simulink model "mod_sim_VTMS"  (R2018b)
settings: Solver=FixedStepDiscrete  StartTime=0.0  StopTime=t_Simulation  FixedStep=delta_t  RelTol=1e-3
values from neighbouring files (symbols this model uses):
  P_charge = 150    [main_sim_VTMS.m]
undefined symbols (not defined in the file or in its folder): A_EMaschine_Getriebe, A_j_c, A_Stirn, Anzahl_Peltierelemente, b_Batteriepack, b_c, b_EMaschine, b_Getriebe, b_j, b_Ladegeraet, BatPara, c_W, delta_t, DiscIntNeverNeededParam, e_Fahrzeug, eta_EMaschine_Break_M_EMaschine, eta_EMaschine_Break_n_EMaschine, eta_EMaschine_Faktor_Volllast, eta_EMaschine_Table, eta_Getriebe, eta_Ladegeraet, eta_Leistungselektronik_Break_M_EMaschine, eta_Leistungselektronik_Break_n_EMaschine, eta_Leistungselektronik_Faktor_Volllast, eta_Leistungselektronik_Table, f_R, I_DT_U_Break_DT, I_DT_U_Break_U, I_DT_U_Value_I, i_Getriebe, I_max, Ladevorgang, M_EMaschine_max, m_Fahrzeug, m_Zuladung, n_Zelle, P_Nebenverbraucher, p_Zelle, Peltier_Max_Eff, Q_DT_U_Break_DT, Q_DT_U_Break_U, Q_DT_U_Value_Q, Q_Imax_DT_Break_DT, Q_Imax_DT_Value_Q, r_dynamisch, rho_Luft, s_Zelle, SOC_init, Steuerung_Kuehlerluefter, Steuerung_Pumpe, Steuerung_Ventil, switch_BP_Zyklus, T_Batteriepack_init, T_EMaschine_Getriebe_init, T_Ladegeraet_init, T_Ladegeraet_Offset, T_Leistungselektronik_init, T_Offset_Batteriepack, T_Offset_EMaschine_Getriebe, T_Offset_Leistungselektronik ... (+36)
libraries: simulink x3, simulink_extras x2
(part 2 of 5)

== system mod_sim_VTMS/Thermomanagementsystem/Schlauch ==
  Fluid_Schlauch_Output : Inport
  T_Umgebung [K] : Inport  Port=2
  v_Fahrzeug [m*s^-1] : Inport  Port=3
  Bus Creator : BusCreator  Inputs=11
  Bus Selector : BusSelector  OutputSignals=T_FinitesVolumen_Schlauch(1) [K],PV_Kuehlfluessigkeit_Schlauch(1) [m^3*s^-1],T_FinitesVolumen_Schlauch(2) [K],PV_Kuehlfluessigkeit_Schlauch(2) [m^3*s^-1],T_FinitesVolumen_Schlauch(3) [K],PV_Kuehlfluessigkeit_Schlauch(3) [m^3*s^-1],T_FinitesVolumen_Schlauch(4) [K],PV_Kuehlfluessigkeit_Schlauch(4) [m^3*s^-1],T_FinitesVolumen_Schlauch(5) [K],PV_Kuehlfluessigkeit_Schlauch(5) [m^3*s^-1],T_FinitesVolumen_Schlauch(6) [K],PV_Kuehlfluessigkeit_Schlauch(6) [m^3*s^-1],T_FinitesVolumen_Schlauch(7) [K],PV_Kuehlfluessigkeit_Schlauch(7) [m^3*s^-1],T_FinitesVolumen_Schlauch(8) [K],PV_Kuehlfluessigkeit_Schlauch(8) [m^3*s^-1],T_FinitesVolumen_Schlauch(9) [K],PV_Kuehlfluessigkeit_Schlauch(9) [m^3*s^-1],T_FinitesVolumen_Schlauch(10) [K],PV_Kuehlfluessigkeit_Schlauch(10) [m^3*s^-1],T_FinitesVolumen_Schlauch(11) [K],PV_Kuehlfluessigkeit_Schlauch(11) [m^3*s^-1]
  Schlauch thermisch : Subsystem
  Schlauch_Output : Outport
  wires:
  Bus Creator/1 -> Schlauch_Output/1
  Fluid_Schlauch_Output/1 -> Bus Selector/1

== system mod_sim_VTMS/Thermomanagementsystem/Wärmetauscher ==
  Fluid_Waermetauscher_Output : Inport
  T_Umgebung [K] : Inport  Port=2
  v_Fahrzeug [m*s^-1] : Inport  Port=3
  Bus Creator : BusCreator  Inputs=2
  Bus Selector : BusSelector  OutputSignals=T_FinitesVolumen_Waermetauscher(1_1) [K],PV_Kuehlfluessigkeit_Waermetauscher(1_1) [m^3*s^-1],T_FinitesVolumen_Waermetauscher(2_1) [K],PV_Kuehlfluessigkeit_Waermetauscher(2_1) [m^3*s^-1]
  Waermetauscher thermisch : Subsystem
  Waermetauscher_Output : Outport
  wires:
  Bus Creator/1 -> Waermetauscher_Output/1
  Fluid_Waermetauscher_Output/1 -> Bus Selector/1

== system mod_sim_VTMS/Thermomanagementsystem/switch_BP_Zyklus ==
  Rad_Output_Zyklus : Inport
  v_Fahrzeug_Zyklus [m/s] : Inport  Port=2
  Rad_Output_BP : Inport  Port=3
  v_Fahrzeug_BP [m/s] : Inport  Port=4
  Constant : Constant  Value=switch_BP_Zyklus
  Switch : Switch  Criteria=u2 ~= 0
  Switch1 : Switch  Criteria=u2 ~= 0
  v_Fahrzeug [m*s^-1] : Outport
  Rad_Output : Outport  Port=2
  wires:
  Constant/1 -> Switch/2, Switch1/2
  Switch1/1 -> v_Fahrzeug [m*s^-1]/1
  Switch/1 -> Rad_Output/1
  v_Fahrzeug_BP [m/s]/1 -> Switch1/1
  v_Fahrzeug_Zyklus [m/s]/1 -> Switch1/3
  Rad_Output_Zyklus/1 -> Switch/3
  Rad_Output_BP/1 -> Switch/1

== system mod_sim_VTMS/Thermomanagementsystem/Batteriepack/Abbruch, wenn SOC <= 0 ==
  SOC_Batteriepack [-] : Inport
  Relational Operator : RelationalOperator  Operator=<=  OutDataTypeStr=boolean  RndMeth=Simplest
  SoC_min [-] : Constant  Value=0
  Stop Simulation : Stop
  wires:
  SoC_min [-]/1 -> Relational Operator/2
  Relational Operator/1 -> Stop Simulation/1
  SOC_Batteriepack [-]/1 -> Relational Operator/1

== system mod_sim_VTMS/Thermomanagementsystem/Batteriepack/Batteriepack(1) elektrisch ==
  note: -> Annahme: Das Batteriepack besteht aus komplett identischen Zellen
      | -> Annahme: Das Batteriepack besteht aus NCR18650PF-Zellen (zylindrische Lithium-Ionen-Zelle)
      | -> Deswegen ist das Batteriepack derart modelliert, dass dass nur eine Zelle elektrisch berechnet wird und basierend auf den resultierenden Zellgrößen die Batteriepackgrößen bestimmt werden
      | -> Dazu ist ein Zellmodell aus dem am FTM vorhandenen Batteriepackmodell, das im Rahmen der Semesterarbeit "Modellbasierte Entwicklung eines vollparametrischen Batteriepackmodells für Elektro- und Hybridfahrzeuge" entwickelt wurde, abgeleitet
      |
      | -> Die Strombelastung einer Zelle wird aus der Leistungsanforderung an eine Zelle und der Klemmenspannung einer Zelle berechnet
      | -> E ine positive Leistungsanforderung an eine Zelle führt zu deren Entladung
      | -> Im Batteriepackmodell bzw. im daraus abgeleiteten Zellmodell sind Entladeströme negativ definiert
      | -> Deswegen wird bei der Berechnung der Strombelastung einer Zelle mit -1 multipliziert, um bei einer positiven Leistungsanforderung an eine Zelle korrekterweise eine negative Strombelastung einer Zelle zu erhalten
      | -> Das Zellmodell berechnet zu einem Auswertungszeitpunkt basierend auf der Strombelastung einer Zelle die Klemmenspannung einer Zelle
      | -> Deswegen muss bei der Berechnung der Strombelastung einer Zelle die Klemmenspannung einer Zelle vom vorherigen Auswertungszeitpunkt verwendet werden
      | -> Dadurch wird ein Fehler gemacht, der wegen der zeitdiskreten Auswertung jedoch nicht vermeidbar ist
      | -> Zu Beginn der Simulation wird statt der Klemmenspannung einer Zelle vom vorherigen Auswertungszeitpunkt das initiale Potential einer Zelle herangezogen
      | -> U_Potential_init = U_SOC_init + U_Hysterese_init + U_RC1_init + U_RC2_init
      |
      | P_Zelle = P_Batteriepack / n_Zelle
      | mit n_Zelle = p_Zelle * s_Zelle
      |
      | I_Zelle = - P_Zelle / U_Zelle
  note: -> Das Batteriepackmodell basiert auf Temperaturen in °C statt in K
      |
      | -> Das Batteriepack wird als Blockkapazität betrachtet
      | -> Temperatur des Batteriepacks = Temperatur jeder Zelle
  T_Batteriepack [K] : Inport
  P_Batteriepack [W] : Inport  Port=2
  Add : Sum  Inputs=++++
  Batteriepackgrößen : Subsystem
  Constant : Constant  Value=SOC_init  VectorParams1D=off
  Constant1 : Constant  Value=U_Hysterese_init  VectorParams1D=off
  Constant2 : Constant  Value=U_RC1_init  VectorParams1D=off
  Constant3 : Constant  Value=U_RC2_init  VectorParams1D=off
  Constant4 : Constant  Value=n_Zelle  VectorParams1D=off
  Constant5 : Constant  Value=273.15  VectorParams1D=off
  Delay : Delay  DelayLength=1  InitialConditionSource=Input port  InitialCondition=0
      settings: InputPortMap=u0,p4
  Divide : Product  Inputs=*/
  Divide1 : Product  Inputs=*/
  Gain : Gain  Gain=-1
  SOC --> U_SOC : Lookup_n-D  NumberOfTableDimensions=1  BreakpointsForDimension1=BatPara.ECMPara.OCV.Steps.SOC_ch  BreakpointsForDimension2=[1:3]  IndexSearchMethod=Linear search  BeginIndexSearchUsingPreviousIndexResult=on  Table=BatPara.ECMPara.OCV.Steps.U_mean  ExtrapMethod=Clip  RemoveProtectionInput=on  UseLastTableValue=on  RndMeth=Simplest  InputSameDT=on
  Subtract : Sum  Inputs=+-
  "Zellmodell (abgeleitet aus Batteriepackmodell -> siehe FTM)" : Subsystem  TreatAsAtomicUnit=on
  I_Batteriepack [A] : Outport
  U_Batteriepack [V] : Outport  Port=2
  SOC_Batteriepack [-] : Outport  Port=3
  eta_Batteriepack [%] : Outport  Port=4
  P_Verlust_Batteriepack [W] : Outport  Port=5
  wires:
  Batteriepackgrößen/4(eta_Batteriepack [%]) -> eta_Batteriepack [%]/1
  Batteriepackgrößen/2(U_Batteriepack [V]) -> U_Batteriepack [V]/1
  Batteriepackgrößen/1(I_Batteriepack [A]) -> I_Batteriepack [A]/1
  Constant5/1 -> Subtract/2
  Subtract/1 -> "Zellmodell (abgeleitet aus Batteriepackmodell -> siehe FTM)"/2(T_Zelle [°C])
  "Zellmodell (abgeleitet aus Batteriepackmodell -> siehe FTM)"/4(P_Verlust_Zelle_reversibel [W]) -> Batteriepackgrößen/6(P_Verlust_Zelle_reversibel [W])
  Add/1 -> Delay/2
  "Zellmodell (abgeleitet aus Batteriepackmodell -> siehe FTM)"/1(U_Zelle [V]) -> Batteriepackgrößen/3(U_Zelle [V]), Delay/1
  Delay/1 -> Divide1/2  "U_Zelle [V]"
  SOC --> U_SOC/1 -> Add/1
  Constant/1 -> SOC --> U_SOC/1
  Divide1/1 -> Gain/1
  Constant1/1 -> Add/2
  Constant4/1 -> Divide/2
  "Zellmodell (abgeleitet aus Batteriepackmodell -> siehe FTM)"/3(P_Verlust_Zelle_irreversibel [W]) -> Batteriepackgrößen/5(P_Verlust_Zelle_irreversibel [W])
  Divide/1 -> Divide1/1, Batteriepackgrößen/1(P_Zelle [W])  "P_Zelle [W]"
  P_Batteriepack [W]/1 -> Divide/1
  Constant2/1 -> Add/3
  Batteriepackgrößen/5(P_Verlust_Batteriepack [W]) -> P_Verlust_Batteriepack [W]/1
  T_Batteriepack [K]/1 -> Subtract/1
  Constant3/1 -> Add/4
  Gain/1 -> "Zellmodell (abgeleitet aus Batteriepackmodell -> siehe FTM)"/1(I_Zelle [A]), Batteriepackgrößen/2(I_Zelle [A])
  "Zellmodell (abgeleitet aus Batteriepackmodell -> siehe FTM)"/2(SOC_Zelle [-]) -> Batteriepackgrößen/4(SOC_Zelle [-])
  Batteriepackgrößen/3("SOC_Batteriepack [-] ") -> SOC_Batteriepack [-]/1

== system mod_sim_VTMS/Thermomanagementsystem/Batteriepack/Batteriepack(1) thermisch ==
  note: T_Batteriepack_k+1 = T_Batteriepack_k + delta_T_Batteriepack für k = Auswertungszeitpunkt
      | = T_Batteriepack_k + b_Batteriepack * (P_Verlust_Batteriepack_k - PQ_Batteriepack_k) für k = Auswertungszeitpunkt
      |
      | mit b_Batteriepack = delta_t / C_Batteriepack
  note: -> Das Batteriepack wird als Blockkapazität aufgefasst und wird nicht als Zusammenschluss einzelner Zellen betrachtet
      |
      | -> Das Batteriepack besitzt eine eigene Temperatur und wird als diabat zu seiner Umgebung betrachtet
      | -> Es gibt also einen Wärmeaustausch zwischen Batteriepack und Umgebungsluft
      | -> Zudem gibt es einen Wärmeaustausch zwischen Batteriepack und Kühlflüssigkeit
      | -> Das Batteriepack besitzt eine Verlustleistung
  P_Verlust_Batteriepack [W] : Inport
  T_FinitesVolumen [K] : Inport  Port=2
  PV_Kuehlfluessigkeit [m^3*s^-1] : Inport  Port=3
  T_Umgebung [K] : Inport  Port=4
  v_Fahrzeug [m*s^-1] : Inport  Port=5
  Add : Sum
  Add1 : Sum
  Add2 : Sum
  Constant : Constant  Value=b_Batteriepack  VectorParams1D=off
  Constant1 : Constant  Value=T_Offset_Batteriepack  VectorParams1D=off
  Product : Product
  Subtract : Sum  Inputs=+-
  Unit Delay : UnitDelay  InitialCondition=T_Batteriepack_init  SampleTime=-1
  Waermeaustausch Batteriepack - Kuehlfluessigkeit : Subsystem
  Waermeaustausch Batteriepack - Umgebungsluft : Subsystem
  T_Batteriepack [K] : Outport
  PQ_Batteriepack_FinitesVolumen [W] : Outport  Port=2
  wires:
  T_FinitesVolumen [K]/1 -> Waermeaustausch Batteriepack - Kuehlfluessigkeit/2(T_FinitesVolumen [K])
  v_Fahrzeug [m*s^-1]/1 -> Waermeaustausch Batteriepack - Umgebungsluft/3(v_Fahrzeug [m*s^-1])
  Add/1 -> Waermeaustausch Batteriepack - Umgebungsluft/2(T_Umgebung_Batteriepack [K])
  Constant1/1 -> Add/2
  T_Umgebung [K]/1 -> Add/1
  Waermeaustausch Batteriepack - Kuehlfluessigkeit/2(PQ_Batteriepack_FinitesVolumen [W]) -> PQ_Batteriepack_FinitesVolumen [W]/1
  Waermeaustausch Batteriepack - Kuehlfluessigkeit/1(PQ_Batteriepack_Kuehlfluessigkeit [W]) -> Add1/2
  Waermeaustausch Batteriepack - Umgebungsluft/1(PQ_Batteriepack_Umgebung [W]) -> Add1/1
  P_Verlust_Batteriepack [W]/1 -> Subtract/1  "P_Verlust_Batteriepack_k [W]"
  Add1/1 -> Subtract/2  "PQ_Batteriepack_k [W]"
  Subtract/1 -> Product/2
  Constant/1 -> Product/1
  Product/1 -> Add2/2  "delta_T_Batteriepack [K]"
  Add2/1 -> Unit Delay/1  "T_Batteriepack_k+1 [K]"
  Unit Delay/1 -> Add2/1, Waermeaustausch Batteriepack - Umgebungsluft/1(T_Batteriepack [K]), Waermeaustausch Batteriepack - Kuehlfluessigkeit/1(T_Batteriepack [K]), T_Batteriepack [K]/1  "T_Batteriepack_k [K]"
  PV_Kuehlfluessigkeit [m^3*s^-1]/1 -> Waermeaustausch Batteriepack - Kuehlfluessigkeit/3(PV_Kuehlfluessigkeit [m^3*s^-1])

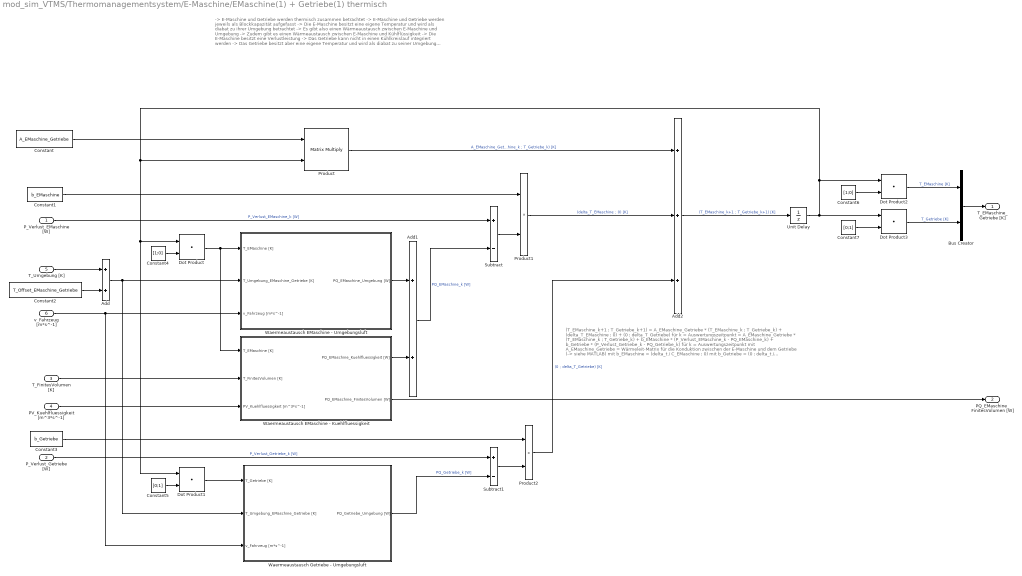
== system mod_sim_VTMS/Thermomanagementsystem/E-Maschine/EMaschine(1) + Getriebe(1) thermisch ==
  note: -> E-Maschine und Getriebe werden thermisch zusammen betrachtet
      | -> E-Maschine und Getriebe werden jeweils als Blockkapazität aufgefasst
      |
      | -> Die E-Maschine besitzt eine eigene Temperatur und wird als diabat zu ihrer Umgebung betrachtet
      | -> Es gibt also einen Wärmeaustausch zwischen E-Maschine und Umgebung
      | -> Zudem gibt es einen Wärmeaustausch zwischen E-Maschine und Kühlflüssigkeit
      | -> Die E-Maschine besitzt eine Verlustleistung
      |
      | -> Das Getriebe kann nicht in einen Kühlkreislauf integriert werden
      | -> Das Getriebe besitzt aber eine eigene Temperatur und wird als diabat zu seiner Umgebung betrachtet
      | -> Es gibt also einen Wärmeaustausch zwischen Umgebung und Getriebe
      | -> Das Getriebe besitzt eine Verlustleistung
      |
      | -> Zwischen E-Maschine und Getriebe findet zudem ein Wärmeaustausch über Konduktion statt
  note: (T_EMaschine_k+1 ; T_Getriebe_k+1) = A_EMaschine_Getriebe * (T_EMaschine_k ; T_Getriebe_k) + (delta_T_EMaschine ; 0) + (0 ; delta_T_Getriebe) für k = Auswertungszeitpunkt
      | 				    				     = A_EMaschine_Getriebe * (T_EMaschine_k ; T_Getriebe_k) + b_EMaschine * (P_Verlust_EMaschine_k - PQ_EMaschine_k) + b_Getriebe * (P_Verlust_Getriebe_k - PQ_Getriebe_k) für k = Auswertungszeitpunkt
      |
      | mit A_EMaschine_Getriebe = Wärmeleit-Matrix für die Konduktion zwischen der E-Maschine und dem Getriebe (-> siehe MATLAB)
      | mit b_EMaschine = (delta_t / C_EMaschine ; 0)
      | mit b_Getriebe = (0 ; delta_t / C_Getriebe)
  P_Verlust_EMaschine [W] : Inport
  P_Verlust_Getriebe [W] : Inport  Port=2
  T_FinitesVolumen [K] : Inport  Port=3
  PV_Kuehlfluessigkeit [m^3*s^-1] : Inport  Port=4
  T_Umgebung [K] : Inport  Port=5
  v_Fahrzeug [m*s^-1] : Inport  Port=6
  Add : Sum
  Add1 : Sum
  Add2 : Sum  Inputs=+++
  Bus Creator : BusCreator  Inputs=2
  Constant : Constant  Value=A_EMaschine_Getriebe  VectorParams1D=off
  Constant1 : Constant  Value=b_EMaschine  VectorParams1D=off
  Constant2 : Constant  Value=T_Offset_EMaschine_Getriebe  VectorParams1D=off
  Constant3 : Constant  Value=b_Getriebe  VectorParams1D=off
  Constant4 : Constant  Value=[1;0]  VectorParams1D=off
  Constant5 : Constant  Value=[0;1]  VectorParams1D=off
  Constant6 : Constant  Value=[1;0]  VectorParams1D=off
  Constant7 : Constant  Value=[0;1]  VectorParams1D=off
  Dot Product{,1..3} (4 alike) : DotProduct  InputSameDT=on  OutDataTypeStr=Inherit: Inherit via internal rule
  Product : Product  Multiplication=Matrix(*)
  Product1 : Product
  Product2 : Product
  Subtract : Sum  Inputs=+-
  Subtract1 : Sum  Inputs=+-
  Unit Delay : UnitDelay  InitialCondition=T_EMaschine_Getriebe_init  SampleTime=-1
  Waermeaustausch EMaschine - Kuehlfluessigkeit : Subsystem
  "Waermeaustausch EMaschine - Umgebungsluft " : Subsystem
  Waermeaustausch Getriebe - Umgebungsluft : Subsystem
  T_EMaschine_Getriebe [K] : Outport
  PQ_EMaschine_FinitesVolumen [W] : Outport  Port=2
  wires:
  Unit Delay/1 -> Product/2, Dot Product/1, Dot Product1/1, Dot Product2/1, Dot Product3/1
  Constant/1 -> Product/1
  Product/1 -> Add2/1  "A_EMaschine_Getriebe * (T_EMaschine_k ; T_Getriebe_k) [K]"
  Add2/1 -> Unit Delay/1  "(T_EMaschine_k+1 ; T_Getriebe_k+1) [K]"
  P_Verlust_EMaschine [W]/1 -> Subtract/1  "P_Verlust_EMaschine_k [W]"
  Add1/1 -> Subtract/2  "PQ_EMaschine_k [W]"
  Constant1/1 -> Product1/1
  Subtract/1 -> Product1/2
  Product1/1 -> Add2/2  "(delta_T_EMaschine ; 0) [K]"
  Constant3/1 -> Product2/1
  Product2/1 -> Add2/3  "(0 ; delta_T_Getriebe) [K]"
  Constant4/1 -> Dot Product/2
  Dot Product/1 -> "Waermeaustausch EMaschine - Umgebungsluft "/1(T_EMaschine [K]), Waermeaustausch EMaschine - Kuehlfluessigkeit/1(T_EMaschine [K])
  Constant5/1 -> Dot Product1/2
  Add/1 -> "Waermeaustausch EMaschine - Umgebungsluft "/2(T_Umgebung_EMaschine_Getriebe [K]), Waermeaustausch Getriebe - Umgebungsluft/2(T_Umgebung_EMaschine_Getriebe [K])
  Dot Product1/1 -> Waermeaustausch Getriebe - Umgebungsluft/1(T_Getriebe [K])
  Constant6/1 -> Dot Product2/2
  Bus Creator/1 -> T_EMaschine_Getriebe [K]/1
  Constant7/1 -> Dot Product3/2
  Dot Product3/1 -> Bus Creator/2  "T_Getriebe [K]"
  Dot Product2/1 -> Bus Creator/1  "T_EMaschine [K]"
  "Waermeaustausch EMaschine - Umgebungsluft "/1(PQ_EMaschine_Umgebung [W]) -> Add1/1
  T_Umgebung [K]/1 -> Add/1
  Constant2/1 -> Add/2
  P_Verlust_Getriebe [W]/1 -> Subtract1/1  "P_Verlust_Getriebe_k [W]"
  Waermeaustausch Getriebe - Umgebungsluft/1(PQ_Getriebe_Umgebung [W]) -> Subtract1/2  "PQ_Getriebe_k [W]"
  Subtract1/1 -> Product2/2
  T_FinitesVolumen [K]/1 -> Waermeaustausch EMaschine - Kuehlfluessigkeit/2(T_FinitesVolumen [K])
  Waermeaustausch EMaschine - Kuehlfluessigkeit/2(PQ_EMaschine_FinitesVolumen [W]) -> PQ_EMaschine_FinitesVolumen [W]/1
  Waermeaustausch EMaschine - Kuehlfluessigkeit/1(PQ_EMaschine_Kuehlfluessigkeit [W]) -> Add1/2
  v_Fahrzeug [m*s^-1]/1 -> "Waermeaustausch EMaschine - Umgebungsluft "/3(v_Fahrzeug [m*s^-1]), Waermeaustausch Getriebe - Umgebungsluft/3(v_Fahrzeug [m*s^-1])
  PV_Kuehlfluessigkeit [m^3*s^-1]/1 -> Waermeaustausch EMaschine - Kuehlfluessigkeit/3(PV_Kuehlfluessigkeit [m^3*s^-1])

== system mod_sim_VTMS/Thermomanagementsystem/Fluid/Bestimmung PV_Kuehlkreislauf ==
  EMaschine_Output : Inport
  Leistungselektronik_Output : Inport  Port=2
  Batteriepack_Output : Inport  Port=3
  Bus Creator : BusCreator  Inputs=2
  Kuehlkreislauf : Subsystem
  PV_Kuehlkreislauf [m^3*s^-1] : Outport
  wires:
  Bus Creator/1 -> PV_Kuehlkreislauf [m^3*s^-1]/1

== system mod_sim_VTMS/Thermomanagementsystem/Fluid/Bestimmung Zustand_Ventil ==
  Fluid_Schlauch_Output : Inport
  Bus Creator : BusCreator  Inputs=1
  Ventil : Subsystem
  Zustand_Ventil [-] : Outport
  wires:
  Bus Creator/1 -> Zustand_Ventil [-]/1

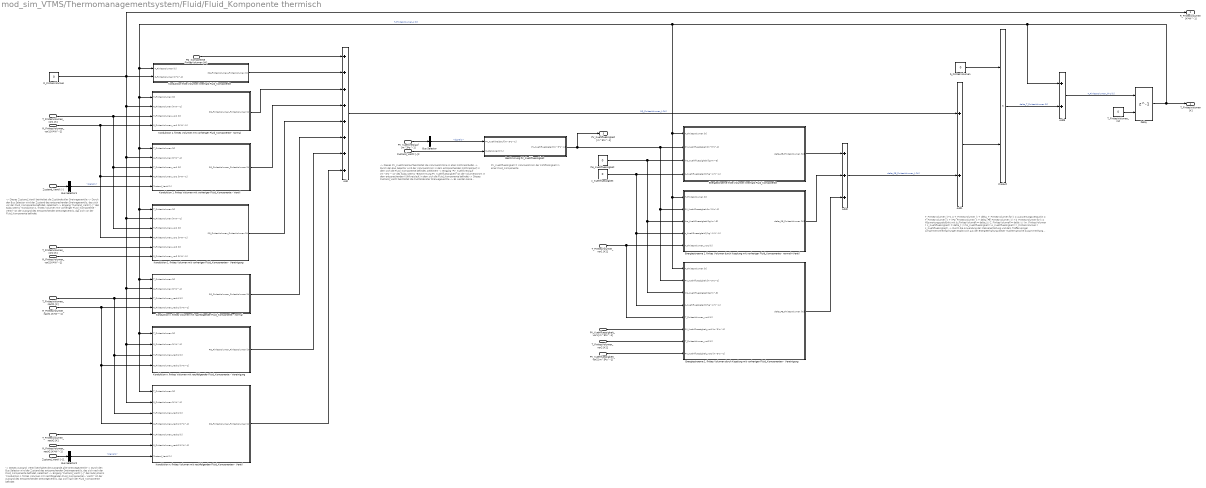
== system mod_sim_VTMS/Thermomanagementsystem/Fluid/Fluid_Komponente thermisch ==
  note: -> Dieses PV_Kuehlkreislauf beinhaltet die Volumenströme in allen Kühlkreisläufen
      | -> Durch den Bus Selector wird der Volumenstrom in dem entsprechenden Kühlkreislauf, in dem sich die Fluid_Komponente befindet, selektiert
      | -> Eingang "PV_Kuehlkreislauf [m^3*s^-1]" des Subsystems "Bestimmung PV_Kuehlfluessigkeit" ist der Volumenstrom in dem entsprechenden Kühlkreislauf, in dem sich die Fluid_Komponente befindet
      |
      | -> Dieses Zustand_Ventil beinhaltet die Zustände aller Dreiwegeventile
      | -> Es werden keine Zustände bestimmter Dreiwegeventile selektiert
      | -> Eingang "Zustand_Ventil [-]" des Subsystems "Bestimmung PV_Kuehlfluessigkeit" ist der Bus mit den Zuständen aller Dreiwegeventile
  note: T_FinitesVolumen_k+1 = T_FinitesVolumen_k + delta_T_FinitesVolumen für k = Auswertungszeitpunkt
      | = T_FinitesVolumen_k + (PQ_FinitesVolumen_k + delta_PE_FinitesVolumen_k) * b_FinitesVolumen für k = Auswertungszeitpunkt
      |
      | mit b_FinitesVolumen = delta_t / C_FinitesVolumen = delta_t / (m_FinitesVolumen * c_Kuehlfluessigkeit) = delta_t / (rho_Kuehlfluessigkeit * A_Kuehlfluessigkeit * l_FinitesVolumen * c_Kuehlfluessigkeit)
      |
      | -> Durch die Anwendung der Massenerhaltung und dem Treffen einiger Annahmen/Vereinfachungen ergibt sich aus der Energieerhaltung dieser mathematische Zusammenhang
      | -> Für die genaue Herleitung wird auf wird auf die im Rahmen des Thermomanagementsystemmodells erstellte Masterarbeit "Entwicklung und Steuerung eines Thermomanagementsystemmodells für Elektrofahrzeuge" verwiesen
      | -> Eine Temperaturänderung der Kühlflüssigkeit bzgl. des Knotens eines finiten Volumens resultiert aus einem Wärmestrom bzgl. des finiten Volumens (Wärmeübertragung zwischen Komponente und Kühlflüssigkeit in finiten Volumen sowie Konduktion mit benachbarten finiten Volumen) PQ_FinitesVolumen und der Differenz der Energieströme zwischen Eingang und Ausgang des finiten Voumens delta_PE_FinitesVolumen
      |
      | -> Örtliche Diskretisierung:
      | -> 1D-Simulation in axialer Richtung -> Strömungsgrößen in einem Kühlkreislauf können sich nur in axialer Richtung örtlich unterscheiden und diese sind jeweils über die gesamte zur axialen Achse senkrecht ausgerichtete Querschnittsfläche örtlich konstant
      | -> Diskretisierung mittels Finite-Volume n-Methode nur in axialer Richtung -> Jedes durch die Diskretisierung resultierende finite Volumen hat die gleiche Länge und seinen Knoten im Mittelpunkt -> Zusätzlich wird ein finites Volumen durch seine zur axialen Achse senkrecht ausgerichtete Querschnittsfläche repräsentiert -> I nnerhalb einer Fluid_Komponente hat jedes finite Volumen die gleiche Querschnittsfläche, aber unterschiedlich zwischen Fluid_Komponenten möglich
      | -> Für jedes finite Volumen wird der Erhaltungssatz der Energie in integraler Form ausgewertet und dadurch die Temperatur des finiten Volumens berechnet
      | -> Für die Interpolation des Wertes einer Größe an der Grenzfläche wird die Aufwind-Interpolation verwendet -> Wert einer Größe an einer Grenzfläche ist identisch dem Wert der Größe im Knoten desjenigen finiten Volumens, dessen Normalenvektor an der betrachteten Grenzfläche mit der Strömungsrichtung übereinstimmt
      | -> Quadratur wird nicht benötigt, weil aufgrund der 1D-Simulation der Wert einer Größe an der Grenzfläche über die gesamte Grenzfläche konstant ist
      |
      | -> Zeitliche Diskretisierung:
      | -> Explizite Euler-Methode -> T_k+1 = T_k + f (Werte der Größen zu k) * delta_t für k = Auswertungszeitpunkt
  note: PV_Kuehlfluessigkeit = Volumenstrom der Kühlflüssigkeit in einer Fluid_Komponente
  note: -> Dieses Zustand_Ventil beinhaltet die Zustände aller Dreiwegeventile
      | -> Durch den Bus Selector wird der Zustand des entsprechenden Dreiwegeventils, das sich vor der Fluid_Komponente befindet, selektiert
      | -> Eingang "Zustand_Ventil [-]" des Subsystems "Konduktion 1. finites Volumen mit vorheriger Fluid_Komponente - Ventil" ist der Zustand des entsprechenden Dreiwegeventils, das sich vor der Fluid_Komponente befindet
  note: -> Dieses Zustand_Ventil beinhaltet die Zustände aller Dreiwegeventile
      | -> Durch den Bus Selector wird der Zustand des entsprechenden Dreiwegeventils, das sich nach der Fluid_Komponente befindet, selektiert
      | -> Eingang "Zustand_Ventil [-]" des Subsystems "Konduktion n. finites Volumen mit nachfolgenden Fluid_Komponenten - Ventil" ist der Zustand des entsprechenden Dreiwegeventils, das sich nach der Fluid_Komponente befindet
  PV_Kuehlkreislauf [m^3*s^-1] : Inport
  PQ_Komponente_FinitesVolumen [W] : Inport  Port=2
  T_FinitesVolumen_vor1 [K] : Inport  Port=3
  R_FinitesVolumen_vor1 [K*W^-1] : Inport  Port=4
  PV_Kuehlfluessigkeit_vor1 [m^3*s^-1] : Inport  Port=5
  T_FinitesVolumen_vor2 [K] : Inport  Port=6
  R_FinitesVolumen_vor2 [K*W^-1] : Inport  Port=7
  PV_Kuehlfluessigkeit_vor2 [m^3*s^-1] : Inport  Port=8
  T_FinitesVolumen_nach1 [K] : Inport  Port=9
  R_FinitesVolumen_nach1 [K*W^-1] : Inport  Port=10
  T_FinitesVolumen_nach2 [K] : Inport  Port=11
  R_FinitesVolumen_nach2 [K*W^-1] : Inport  Port=12
  Zustand_Ventil [-] : Inport  Port=13
  Add : Sum  Inputs=++++++++
  Add1 : Sum
  Add2 : Sum  Inputs=+++
  Add3 : Sum
  Bestimmung PV_Kuehlfluessigkeit : Subsystem
  Bus Selector : BusSelector  OutputSignals=signal1
  Bus Selector1 : BusSelector  OutputSignals=signal1
  Bus Selector2 : BusSelector  OutputSignals=signal1
  Delay : Delay  DelayLength=1  InitialConditionSource=Input port  InitialCondition=0
      settings: InputPortMap=u0,p4
  Energiestroeme 1. finites Volumen durch Kopplung mit vorherigen Fluid_Komponenten - Vereinigung : Subsystem
  Energiestroeme 1. finites Volumen durch Kopplung mit vorheriger Fluid_Komponente - normal+Ventil : Subsystem
  Energiestroeme finite Volumen innerhalb Fluid_Komponente : Subsystem
  Konduktion 1. finites Volumen mit vorherigen Fluid_Komponenten - Vereinigung : Subsystem
  Konduktion 1. finites Volumen mit vorheriger Fluid_Komponente - Ventil : Subsystem
  Konduktion 1. finites Volumen mit vorheriger Fluid_Komponente - normal : Subsystem
  Konduktion finite Volumen innerhalb Fluid_Komponente : Subsystem
  Konduktion n. finites Volumen mit nachfolgenden Fluid_Komponenten - Ventil : Subsystem
  Konduktion n. finites Volumen mit nachfolgender Fluid_Komponente - Vereinigung : Subsystem
  Konduktion n. finites Volumen mit nachfolgender Fluid_Komponente - normal : Subsystem
  Product : Product
  R_FinitesVolumen : Constant  Value=0  VectorParams1D=off
  T_FinitesVolumen_init : Constant  Value=0  VectorParams1D=off
  T_FinitesVolumen_vor1 [K]1 : InportShadow  Port=3
  T_FinitesVolumen_vor2 [K]1 : InportShadow  Port=6
  Zustand_Ventil [-]1 : InportShadow  Port=13
  Zustand_Ventil [-]2 : InportShadow  Port=13
  b_FinitesVolumen : Constant  Value=0  VectorParams1D=off
  c_Kuehlfluessigkeit : Constant  Value=0  VectorParams1D=off
  rho_Kuehlfluessigkeit : Constant  Value=0  VectorParams1D=off
  T_FinitesVolumen [K] : Outport
  R_FinitesVolumen [K*W^-1] : Outport  Port=2
  PV_Kuehlfluessigkeit [m^3*s^-1] : Outport  Port=3
  wires:
  Konduktion finite Volumen innerhalb Fluid_Komponente/1(PQ_FinitesVolumen_FinitesVolumen [W]) -> Add/2
  PQ_Komponente_FinitesVolumen [W]/1 -> Add/1
  T_FinitesVolumen_init/1 -> Delay/2
  R_FinitesVolumen/1 -> Konduktion n. finites Volumen mit nachfolgenden Fluid_Komponenten - Ventil/2(R_FinitesVolumen [K*W^-1]), Konduktion n. finites Volumen mit nachfolgender Fluid_Komponente - Vereinigung/2(R_FinitesVolumen [K*W^-1]), Konduktion n. finites Volumen mit nachfolgender Fluid_Komponente - normal/2(R_FinitesVolumen [K*W^-1]), Konduktion 1. finites Volumen mit vorherigen Fluid_Komponenten - Vereinigung/2(R_FinitesVolumen [K*W^-1]), Konduktion 1. finites Volumen mit vorheriger Fluid_Komponente - Ventil/2(R_FinitesVolumen [K*W^-1]), Konduktion 1. finites Volumen mit vorheriger Fluid_Komponente - normal/2(R_FinitesVolumen [K*W^-1]), Konduktion finite Volumen innerhalb Fluid_Komponente/2(R_FinitesVolumen [K*W^-1]), R_FinitesVolumen [K*W^-1]/1
  T_FinitesVolumen_nach1 [K]/1 -> Konduktion n. finites Volumen mit nachfolgenden Fluid_Komponenten - Ventil/3(T_FinitesVolumen_nach1 [K]), Konduktion n. finites Volumen mit nachfolgender Fluid_Komponente - Vereinigung/3(T_FinitesVolumen_nach1 [K]), Konduktion n. finites Volumen mit nachfolgender Fluid_Komponente - normal/3(T_FinitesVolumen_nach1 [K])
  R_FinitesVolumen_nach1 [K*W^-1]/1 -> Konduktion n. finites Volumen mit nachfolgenden Fluid_Komponenten - Ventil/4(R_FinitesVolumen_nach1 [K*W^-1]), Konduktion n. finites Volumen mit nachfolgender Fluid_Komponente - Vereinigung/4(R_FinitesVolumen_nach1 [K*W^-1]), Konduktion n. finites Volumen mit nachfolgender Fluid_Komponente - normal/4(R_FinitesVolumen_nach1 [K*W^-1])
  R_FinitesVolumen_nach2 [K*W^-1]/1 -> Konduktion n. finites Volumen mit nachfolgenden Fluid_Komponenten - Ventil/6(R_FinitesVolumen_nach2 [K*W^-1])
  T_FinitesVolumen_nach2 [K]/1 -> Konduktion n. finites Volumen mit nachfolgenden Fluid_Komponenten - Ventil/5(T_FinitesVolumen_nach2 [K])
  R_FinitesVolumen_vor1 [K*W^-1]/1 -> Konduktion 1. finites Volumen mit vorherigen Fluid_Komponenten - Vereinigung/4(R_FinitesVolumen_vor1 [K*W^-1]), Konduktion 1. finites Volumen mit vorheriger Fluid_Komponente - Ventil/4(R_FinitesVolumen_vor1 [K*W^-1]), Konduktion 1. finites Volumen mit vorheriger Fluid_Komponente - normal/4(R_FinitesVolumen_vor1 [K*W^-1])
  T_FinitesVolumen_vor1 [K]/1 -> Konduktion 1. finites Volumen mit vorherigen Fluid_Komponenten - Vereinigung/3(T_FinitesVolumen_vor1 [K]), Konduktion 1. finites Volumen mit vorheriger Fluid_Komponente - Ventil/3(T_FinitesVolumen_vor1 [K]), Konduktion 1. finites Volumen mit vorheriger Fluid_Komponente - normal/3(T_FinitesVolumen_vor1 [K])
  Bus Selector1/1 -> Konduktion 1. finites Volumen mit vorheriger Fluid_Komponente - Ventil/5(Zustand_Ventil [-])  "<signal1>"
  R_FinitesVolumen_vor2 [K*W^-1]/1 -> Konduktion 1. finites Volumen mit vorherigen Fluid_Komponenten - Vereinigung/6(R_FinitesVolumen_vor2 [K*W^-1])
  T_FinitesVolumen_vor2 [K]/1 -> Konduktion 1. finites Volumen mit vorherigen Fluid_Komponenten - Vereinigung/5(T_FinitesVolumen_vor2 [K])
  Bus Selector2/1 -> Konduktion n. finites Volumen mit nachfolgenden Fluid_Komponenten - Ventil/7(Zustand_Ventil [-])  "<signal1>"
  Konduktion 1. finites Volumen mit vorheriger Fluid_Komponente - normal/1(PQ_FinitesVolumen_FinitesVolumen [W]) -> Add/3
  Konduktion 1. finites Volumen mit vorheriger Fluid_Komponente - Ventil/1(PQ_FinitesVolumen_FinitesVolumen [W]) -> Add/4
  Konduktion 1. finites Volumen mit vorherigen Fluid_Komponenten - Vereinigung/1(PQ_FinitesVolumen_FinitesVolumen [W]) -> Add/5
  Konduktion n. finites Volumen mit nachfolgender Fluid_Komponente - normal/1(PQ_FinitesVolumen_FinitesVolumen [W]) -> Add/6
  Konduktion n. finites Volumen mit nachfolgender Fluid_Komponente - Vereinigung/1(PQ_FinitesVolumen_FinitesVolumen [W]) -> Add/7
  Konduktion n. finites Volumen mit nachfolgenden Fluid_Komponenten - Ventil/1(PQ_FinitesVolumen_FinitesVolumen [W]) -> Add/8
  Energiestroeme finite Volumen innerhalb Fluid_Komponente/1(delta_PE_FinitesVolumen [W]) -> Add2/1
  Delay/1 -> T_FinitesVolumen [K]/1, Konduktion n. finites Volumen mit nachfolgenden Fluid_Komponenten - Ventil/1(T_FinitesVolumen [K]), Konduktion n. finites Volumen mit nachfolgender Fluid_Komponente - Vereinigung/1(T_FinitesVolumen [K]), Konduktion n. finites Volumen mit nachfolgender Fluid_Komponente - normal/1(T_FinitesVolumen [K]), Konduktion 1. finites Volumen mit vorherigen Fluid_Komponenten - Vereinigung/1(T_FinitesVolumen [K]), Konduktion 1. finites Volumen mit vorheriger Fluid_Komponente - Ventil/1(T_FinitesVolumen [K]), Konduktion 1. finites Volumen mit vorheriger Fluid_Komponente - normal/1(T_FinitesVolumen [K]), Konduktion finite Volumen innerhalb Fluid_Komponente/1(T_FinitesVolumen [K]), Energiestroeme finite Volumen innerhalb Fluid_Komponente/1(T_FinitesVolumen [K]), Energiestroeme 1. finites Volumen durch Kopplung mit vorherigen Fluid_Komponenten - Vereinigung/1(T_FinitesVolumen [K]), Energiestroeme 1. finites Volumen durch Kopplung mit vorheriger Fluid_Komponente - normal+Ventil/1(T_FinitesVolumen [K]), Add3/1  "T_FinitesVolumen_k [K]"
  Energiestroeme 1. finites Volumen durch Kopplung mit vorheriger Fluid_Komponente - normal+Ventil/1(delta_PE_FinitesVolumen [W]) -> Add2/2
  Energiestroeme 1. finites Volumen durch Kopplung mit vorherigen Fluid_Komponenten - Vereinigung/1(delta_PE_FinitesVolumen [W]) -> Add2/3
  Bus Selector/1 -> Bestimmung PV_Kuehlfluessigkeit/1(PV_Kuehlkreislauf [m^3*s^-1])  "<signal1>"
  rho_Kuehlfluessigkeit/1 -> Energiestroeme finite Volumen innerhalb Fluid_Komponente/3(rho_Kuehlfluessigkeit [kg*m^-3]), Energiestroeme 1. finites Volumen durch Kopplung mit vorherigen Fluid_Komponenten - Vereinigung/3(rho_Kuehlfluessigkeit [kg*m^-3]), Energiestroeme 1. finites Volumen durch Kopplung mit vorheriger Fluid_Komponente - normal+Ventil/3(rho_Kuehlfluessigkeit [kg*m^-3])
  c_Kuehlfluessigkeit/1 -> Energiestroeme finite Volumen innerhalb Fluid_Komponente/4(c_Kuehlfluessigkeit [J*kg^-1*K^-1]), Energiestroeme 1. finites Volumen durch Kopplung mit vorherigen Fluid_Komponenten - Vereinigung/4(c_Kuehlfluessigkeit [J*kg^-1*K^-1]), Energiestroeme 1. finites Volumen durch Kopplung mit vorheriger Fluid_Komponente - normal+Ventil/4(c_Kuehlfluessigkeit [J*kg^-1*K^-1])
  T_FinitesVolumen_vor1 [K]1/1 -> Energiestroeme 1. finites Volumen durch Kopplung mit vorherigen Fluid_Komponenten - Vereinigung/5(T_FinitesVolumen_vor1 [K]), Energiestroeme 1. finites Volumen durch Kopplung mit vorheriger Fluid_Komponente - normal+Ventil/5(T_FinitesVolumen_vor1 [K])
  PV_Kuehlfluessigkeit_vor1 [m^3*s^-1]/1 -> Energiestroeme 1. finites Volumen durch Kopplung mit vorherigen Fluid_Komponenten - Vereinigung/6(PV_Kuehlfluessigkeit_vor1 [m^3*s^-1])
  T_FinitesVolumen_vor2 [K]1/1 -> Energiestroeme 1. finites Volumen durch Kopplung mit vorherigen Fluid_Komponenten - Vereinigung/7(T_FinitesVolumen_vor2 [K])
  PV_Kuehlfluessigkeit_vor2 [m^3*s^-1]/1 -> Energiestroeme 1. finites Volumen durch Kopplung mit vorherigen Fluid_Komponenten - Vereinigung/8(PV_Kuehlfluessigkeit_vor2 [m^3*s^-1])
  Add/1 -> Add1/1  "PQ_FinitesVolumen_k [W]"
  Add2/1 -> Add1/2  "delta_PE_FinitesVolumen_k [W]"
  b_FinitesVolumen/1 -> Product/1
  Add1/1 -> Product/2
  Product/1 -> Add3/2  "delta_T_FinitesVolumen [K]"
  Add3/1 -> Delay/1  "T_FinitesVolumen_k+1 [K]"
  Bestimmung PV_Kuehlfluessigkeit/1(PV_Kuehlfluessigkeit [m^3*s^-1]) -> PV_Kuehlfluessigkeit [m^3*s^-1]/1, Energiestroeme 1. finites Volumen durch Kopplung mit vorherigen Fluid_Komponenten - Vereinigung/2(PV_Kuehlfluessigkeit [m^3*s^-1]), Energiestroeme 1. finites Volumen durch Kopplung mit vorheriger Fluid_Komponente - normal+Ventil/2(PV_Kuehlfluessigkeit [m^3*s^-1]), Energiestroeme finite Volumen innerhalb Fluid_Komponente/2(PV_Kuehlfluessigkeit [m^3*s^-1])
  PV_Kuehlkreislauf [m^3*s^-1]/1 -> Bus Selector/1
  Zustand_Ventil [-]/1 -> Bus Selector1/1
  Zustand_Ventil [-]1/1 -> Bus Selector2/1
  Zustand_Ventil [-]2/1 -> Bestimmung PV_Kuehlfluessigkeit/2(Zustand_Ventil [-])

== system mod_sim_VTMS/Thermomanagementsystem/Kühler/Kuehler thermisch ==
  note: v_Kuehlerluefter = Luftgeschwindigkeit eines Kühlerlüfters
  note: -> Ein Kühler besitzt keine eigene Temperatur, wird aber als diabat zu seiner Umgebung betrachtet
      | -> Es gibt also einen Wärmeaustausch zwischen Umgebungsluft und Kühlflüssigkeit
  note: PQ_Kuehler_FinitesVolumen_i = UA_Kuehler_FinitesVolumen * (T_Umgebung - T_FinitesVolumen_i) für i = 1:n
      |
      | mit UA_Kuehler_FinitesVolumen = f (PV_Kuehlfluessigkeit, v_Kuehlerluefter, v_Fahrzeug)
      |
      | -> UA_Kuehler_FinitesVolumen ist für jedes finite Volumen des Strömungsgebiets eines Kühlers identisch, weil das Strömungsgebiet eines Kühlers durch identische finite Volumen örtlich diskretisiert ist, weil im gesamten Strömungsgebiet eines Kühlers der gleiche Volumenstrom der Kühlflüssigkeit vorliegt und weil ein Kühler gleichmäßig mit einem Luftstrom beaufschlagt wird
      | -> T_Umgebung ist für jedes finite Volumen des Strömungsgebiets eines Kühlers identisch, weil die Temperatur der Umgebungsluft zeitlich und örtlich konstant ist
  T_FinitesVolumen [K] : Inport
  PV_Kuehlfluessigkeit [m^3*s^-1] : Inport  Port=2
  T_Umgebung [K] : Inport  Port=3
  v_Fahrzeug [m*s^-1] : Inport  Port=4
  Bestimmung v_Kuehlerluefter : Subsystem
  Product : Product
  Subtract : Sum  Inputs=+-
  n-D Lookup Table : Lookup_n-D  NumberOfTableDimensions=3  BreakpointsForDimension1=0  BreakpointsForDimension2=0  BreakpointsForDimension3=0  BeginIndexSearchUsingPreviousIndexResult=on  Table=0  ExtrapMethod=Clip  UseLastTableValue=on  InternalRulePriority=Speed  RndMeth=Simplest  InputSameDT=on
  PQ_Kuehler_FinitesVolumen [W] : Outport
  v_Kuehlerluefter [m*s^-1] : Outport  Port=2
  wires:
  PV_Kuehlfluessigkeit [m^3*s^-1]/1 -> n-D Lookup Table/1
  Subtract/1 -> Product/2
  n-D Lookup Table/1 -> Product/1  "UA_Kuehler_FinitesVolumen [W*K^-1]"
  v_Fahrzeug [m*s^-1]/1 -> n-D Lookup Table/3
  Product/1 -> PQ_Kuehler_FinitesVolumen [W]/1
  T_Umgebung [K]/1 -> Subtract/1
  T_FinitesVolumen [K]/1 -> Subtract/2, Bestimmung v_Kuehlerluefter/1(T_FinitesVolumen [K])
  Bestimmung v_Kuehlerluefter/1(v_Kuehlerluefter [m*s^-1]) -> n-D Lookup Table/2, v_Kuehlerluefter [m*s^-1]/1

== system mod_sim_VTMS/Thermomanagementsystem/Ladegeraet/Ladegeraet(1) elektrisch ==
  note: -> Der Start des Ladevorgangs wird über ein Signal gesteuert, das die Werte logisch wahr oder logisch falsch annehmen kann.
      | -> Abhängig vom aktuellen SOC wird über einen 1-D Lookup Table der Ladestrom vorgegeben
      | -> Die Ladeleistung ergibt sich aus der Multiplikation mit der aktuellen Batteriespannung
      | -> Die tatsächliche Ladeleistung ergibt sich aus der Multiplikation mit dem Wirkungsgrad
      | -> Die Verlustleistung ist die Differenz aus Eingangs- und Ausgangsleistung und wird an das thermische System des Ladegeräts weitergeleitet
      |
      | -> Wird ein SOC von 0.999 erreicht wird die Simulation unterbrochen, da der Ladevorgang beendet ist.
  Batteriepack_Output : Inport
  Steuerungssignal : Inport  Port=2
  AND : Logic  IconShape=distinctive  AllPortsSameDT=off  OutDataTypeStr=boolean
  Add : Sum  Inputs=-+
  Bus Selector1 : BusSelector  OutputSignals=SOC_Batteriepack [-],U_Batteriepack [V]
  Compare To Constant : simulink/Logic and Bit Operations/Compare To Constant  relop=<  const=0.98  OutDataTypeStr=boolean
  Fast charging control : Subsystem  TreatAsAtomicUnit=on
  Gain : Gain  Gain=eta_Ladegeraet
  Gain1 : Gain  Gain=1/s_Zelle
  Leistung_Ladegeraet_Bat [W] : Outport
  Verlustleistung_Ladegeraet [W] : Outport  Port=2
  wires:
  Batteriepack_Output/1 -> Bus Selector1/1
  Bus Selector1/1 -> Compare To Constant/1  "<SOC_Batteriepack [-]>"
  Bus Selector1/2 -> Gain1/1  "<U_Batteriepack [V]>"
  Add/1 -> Verlustleistung_Ladegeraet [W]/1
  Gain/1 -> Add/1, Leistung_Ladegeraet_Bat [W]/1
  Fast charging control/1(charging power [W]) -> Gain/1, Add/2
  Steuerungssignal/1 -> AND/1
  Compare To Constant/1 -> AND/2
  AND/1 -> Fast charging control/Enable
  Gain1/1 -> Fast charging control/1(U_cell [V])

== system mod_sim_VTMS/Thermomanagementsystem/Ladegeraet/Ladegeraet(1) thermisch ==
  note: T_Ladegeraet_k+1 = T_Ladegeraet_k + dT_Ladegeraet für k = Auswertungszeitpunkt
      | = T_Ladegeraet_k + (P_Verlust_Ladegeraet_k - PQ_Ladegeraet_k) * b_Ladegeraet für k = Auswertungszeitpunkt
      |
      | mit b_Ladegeraet = dt / C_Ladegeraet
  note: -> Das Ladegeraet ist auf eine Punktmasse reduziert
      |
      | -> Das Ladegeraet besitzt eine eigene Temperatur und wird als diabat zu seiner Umgebung betrachtet
      | -> Es gibt also einen Wärmeaustausch zwischen Ladegeraet und Umgebung
      | -> Zudem gibt es einen Wärmeaustausch zwischen Ladegeraet und Fluid
      | -> Das Ladegeraet besitzt eine Verlustleistung
  P_Verlust_Ladegeraet [W] : Inport
  T_FinitesVolumen [K] : Inport  Port=2
  PV_Kuehlfluessigkeit [m^3*s^-1] : Inport  Port=3
  T_Umgebung [K] : Inport  Port=4
  v_Fahrzeug [m*s^-1] : Inport  Port=5
  Add : Sum
  Add1 : Sum
  Add2 : Sum
  Constant : Constant  Value=b_Ladegeraet  VectorParams1D=off
  Constant1 : Constant  Value=T_Ladegeraet_Offset  VectorParams1D=off
  Product : Product
  Subtract : Sum  Inputs=+-
  Unit Delay : UnitDelay  InitialCondition=T_Ladegeraet_init  SampleTime=-1
  Waermeaustausch Ladegeraet - Fluid : Subsystem
  "Waermeaustausch Ladegeraet - Umgebung " : Subsystem
  T_Ladegeraet [K] : Outport
  PQ_Ladegeraet_FinitesVolumen [W] : Outport  Port=2
  wires:
  T_FinitesVolumen [K]/1 -> Waermeaustausch Ladegeraet - Fluid/2(T_FinitesVolumen [K])
  v_Fahrzeug [m*s^-1]/1 -> "Waermeaustausch Ladegeraet - Umgebung "/3(v_Fahrzeug [m*s^-1])
  Add/1 -> "Waermeaustausch Ladegeraet - Umgebung "/2(T_Umgebung_Offset [K])
  Constant1/1 -> Add/2
  T_Umgebung [K]/1 -> Add/1
  Waermeaustausch Ladegeraet - Fluid/2(PQ_Ladegeraet_FinitesVolumen [W]) -> PQ_Ladegeraet_FinitesVolumen [W]/1
  Waermeaustausch Ladegeraet - Fluid/1(PQ_Ladegeraet_Kuehlfluessigkeit [W]) -> Add1/2
  "Waermeaustausch Ladegeraet - Umgebung "/1(PQ_Ladegeraet_Umgebung [W]) -> Add1/1
  P_Verlust_Ladegeraet [W]/1 -> Subtract/1  "P_Verlust_Ladegeraet_k [W]"
  Add1/1 -> Subtract/2  "PQ_Ladegeraet_k [W]"
  Subtract/1 -> Product/2
  Constant/1 -> Product/1
  Product/1 -> Add2/2  "dT_Ladegeraet [K]"
  Add2/1 -> Unit Delay/1  "T_Ladegeraet_k+1 [K]"
  Unit Delay/1 -> Add2/1, "Waermeaustausch Ladegeraet - Umgebung "/1(T_Ladegeraet [K]), Waermeaustausch Ladegeraet - Fluid/1(T_Ladegeraet [K]), T_Ladegeraet [K]/1  "T_Ladegeraet_k [K]"
  PV_Kuehlfluessigkeit [m^3*s^-1]/1 -> Waermeaustausch Ladegeraet - Fluid/3(PV_Ladegeraet [m^3*s^-1])

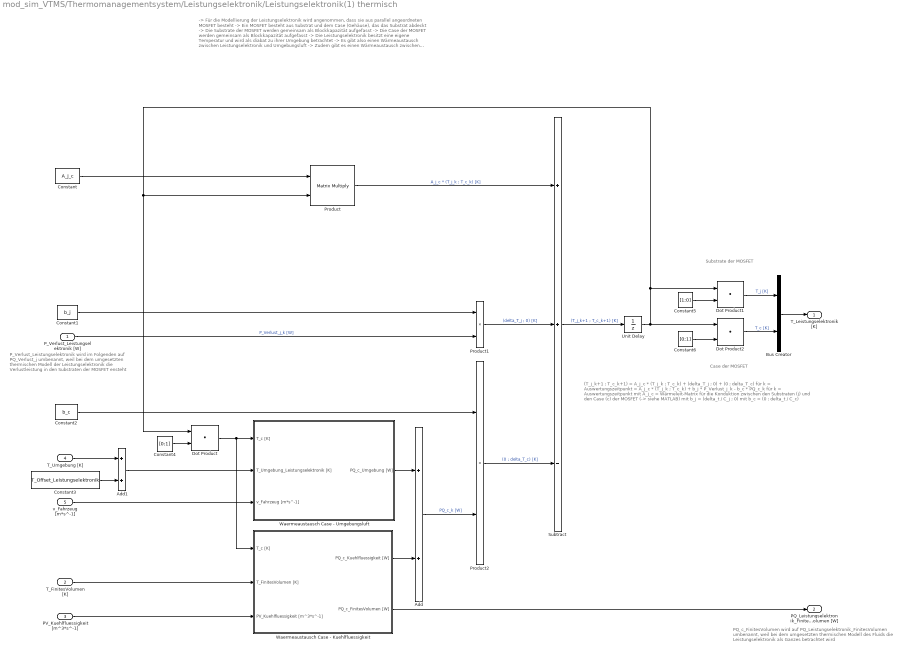
== system mod_sim_VTMS/Thermomanagementsystem/Leistungselektronik/Leistungselektronik(1) thermisch ==
  note: PQ_c_FinitesVolumen wird auf PQ_Leistungselektronik_FinitesVolumen umbenannt, weil bei dem umgesetzten thermischen Modell des Fluids die Leistungselektronik als Ganzes betrachtet wird
  note: -> Für die Modellierung der Leistungselektronik wird angenommen, dass sie aus parallel angeordneten MOSFET besteht
      | -> Ein MOSFET besteht aus Substrat und dem Case (Gehäuse), das das Substrat abdeckt
      | -> Die Substrate der MOSFET werden gemeinsam als Blockkapazität aufgefasst
      | -> Die Case der MOSFET werden gemeinsam als Blockkapazität aufgefasst
      |
      | -> Die Leistungselektronik besitzt eine eigene Temperatur und wird als diabat zu ihrer Umgebung betrachtet
      | -> Es gibt also einen Wärmeaustausch zwischen Leistungselektronik und Umgebungsluft
      | -> Zudem gibt es einen Wärmeaustausch zwischen Leistungselektronik und Kühlflüssigkeit
      | -> Die Leistungselektronik besitzt eine Verlustleistung
      |
      | -> Beide genannten Wärmeaustausche finden über die Case der MOSFET statt
      | -> Die Verlustleistung entsteht in den Substraten der MOSFET
      | -> Zwischen den Substraten und den Case der MOSFET findet zudem eine Wärmeaustausch über Konduktion statt
      | -> Im Thermomanagementsystemmodell sind die Substrate der MOSFET mit j und die Case der MOSFET mit c bezeichnet
  note: Substrate der MOSFET
  note: Case der MOSFET
  note: (T_j_k+1 ; T_c_k+1) = A_j_c * (T_j_k ; T_c_k) + (delta_T_j ; 0) + (0 ; delta_T_c)  für k = Auswertungszeitpunkt
      | 				     = A_j_c * (T_j_k ; T_c_k) + b_j * P_Verlust_j_k - b_c * PQ_c_k  für k = Auswertungszeitpunkt
      |
      | mit A_j_c = Wärmeleit-Matrix für die Konduktion zwischen den Substraten (j) und den Case (c) der MOSFET (-> siehe MATLAB)
      | mit b_j = (delta_t / C_j ; 0)
      | mit b_c = (0 ; delta_t / C_c)
  note: P_Verlust_Leistungselektronik wird im Folgenden auf PQ_Verlust_j umbenannt, weil bei dem umgesetzten thermischen Modell der Leistungselektronik die Verlustleistung in den Substraten der MOSFET ensteht
  P_Verlust_Leistungselektronik [W] : Inport
  T_FinitesVolumen [K] : Inport  Port=2
  PV_Kuehlfluessigkeit [m^3*s^-1] : Inport  Port=3
  T_Umgebung [K] : Inport  Port=4
  v_Fahrzeug [m*s^-1] : Inport  Port=5
  Add : Sum
  Add1 : Sum
  Bus Creator : BusCreator  Inputs=2
  Constant : Constant  Value=A_j_c  VectorParams1D=off
  Constant1 : Constant  Value=b_j  VectorParams1D=off
  Constant2 : Constant  Value=b_c  VectorParams1D=off
  Constant3 : Constant  Value=T_Offset_Leistungselektronik  VectorParams1D=off
  Constant4 : Constant  Value=[0;1]  VectorParams1D=off
  Constant5 : Constant  Value=[1;0]  VectorParams1D=off
  Constant6 : Constant  Value=[0;1]  VectorParams1D=off
  Dot Product : DotProduct  InputSameDT=on  OutDataTypeStr=Inherit: Inherit via internal rule
  Dot Product1 : DotProduct  InputSameDT=on  OutDataTypeStr=Inherit: Inherit via internal rule
  Dot Product2 : DotProduct  InputSameDT=on  OutDataTypeStr=Inherit: Inherit via internal rule
  Product : Product  Multiplication=Matrix(*)
  Product1 : Product
  Product2 : Product
  Subtract : Sum  Inputs=++-
  Unit Delay : UnitDelay  InitialCondition=T_Leistungselektronik_init  SampleTime=-1
  Waermeaustausch Case - Kuehlfluessigkeit : Subsystem
  Waermeaustausch Case - Umgebungsluft : Subsystem
  T_Leistungselektronik [K] : Outport
  PQ_Leistungselektronik_FinitesVolumen [W] : Outport  Port=2
  wires:
  Dot Product1/1 -> Bus Creator/1  "T_j [K]"
  Dot Product2/1 -> Bus Creator/2  "T_c [K]"
  Bus Creator/1 -> T_Leistungselektronik [K]/1
  Unit Delay/1 -> Product/2, Dot Product/1, Dot Product1/1, Dot Product2/1
  Constant/1 -> Product/1
  Constant1/1 -> Product1/1
  P_Verlust_Leistungselektronik [W]/1 -> Product1/2  "P_Verlust_j_k [W]"
  Product/1 -> Subtract/1  "A_j_c * (T_j_k ; T_c_k) [K]"
  Product1/1 -> Subtract/2  "(delta_T_j ; 0) [K]"
  Constant4/1 -> Dot Product/2
  Constant2/1 -> Product2/1
  Constant5/1 -> Dot Product1/2
  Constant6/1 -> Dot Product2/2
  Dot Product/1 -> Waermeaustausch Case - Umgebungsluft/1(T_c [K]), Waermeaustausch Case - Kuehlfluessigkeit/1(T_c [K])
  Add/1 -> Product2/2  "PQ_c_k [W]"
  Waermeaustausch Case - Umgebungsluft/1(PQ_c_Umgebung [W]) -> Add/1
  T_FinitesVolumen [K]/1 -> Waermeaustausch Case - Kuehlfluessigkeit/2(T_FinitesVolumen [K])
  Product2/1 -> Subtract/3  "(0 ; delta_T_c) [K]"
  T_Umgebung [K]/1 -> Add1/1
  Constant3/1 -> Add1/2
  Add1/1 -> Waermeaustausch Case - Umgebungsluft/2(T_Umgebung_Leistungselektronik [K])
  Subtract/1 -> Unit Delay/1  "(T_j_k+1 ; T_c_k+1) [K]"
  Waermeaustausch Case - Kuehlfluessigkeit/2(PQ_c_FinitesVolumen [W]) -> PQ_Leistungselektronik_FinitesVolumen [W]/1
  Waermeaustausch Case - Kuehlfluessigkeit/1(PQ_c_Kuehlfluessigkeit [W]) -> Add/2
  v_Fahrzeug [m*s^-1]/1 -> Waermeaustausch Case - Umgebungsluft/3(v_Fahrzeug [m*s^-1])
  PV_Kuehlfluessigkeit [m^3*s^-1]/1 -> Waermeaustausch Case - Kuehlfluessigkeit/3(PV_Kuehlfluessigkeit [m^3*s^-1])

== system mod_sim_VTMS/Thermomanagementsystem/PCM/PCM thermisch ==
  note: T_PCM_k+1 = T_PCM_k + dT_PCM * Faktor_PW für k = Auswertungszeitpunkt
      | = T_PCM_k - PQ_PCM_k * b_PCM für k = Auswertungszeitpunkt
      |
      | mit b_PCM = dt / C_PCM
  T_FinitesVolumen [K] : Inport
  PV_Kuehlfluessigkeit [m^3*s^-1] : Inport  Port=2
  T_Umgebung [K] : Inport  Port=3
  v_Fahrzeug [m*s^-1] : Inport  Port=4
  Add3 : Sum
  Add4 : Sum
  Add5 : Sum
  Constant16 : Constant  Value=0
  Delay : Delay  DelayLength=1  InitialConditionSource=Input port  InitialCondition=0
      settings: InputPortMap=u0,p4
  PCM_Trigger : FromWorkspace  VariableName=PCM_Trigger  SampleTime=0  OutputAfterFinalValue=Setting to zero
  Phasenuebergang : Subsystem
  Product3 : Product
  Subtract : Sum  Inputs=+-
  T_PCM_Offset : Constant  Value=0  VectorParams1D=off
  T_PCM_init : Constant  Value=273.15  VectorParams1D=off
  Trigger : Subsystem
  Waermeaustausch PCM - Fluid : Subsystem
  Waermeaustausch PCM - Umgebung : Subsystem
  b_PCM : Constant  Value=1.9172735215444e-07  VectorParams1D=off
  T_PCM [K] : Outport
  PQ_PCM_FinitesVolumen [W] : Outport  Port=2
  wires:
  Add3/1 -> Waermeaustausch PCM - Umgebung/2(T_Umgebung_Offset [K])
  Trigger/1(Temp_out) -> Delay/1
  b_PCM/1 -> Product3/1
  Add4/1 -> Subtract/2  "PQ_PCM_k [W]"
  T_Umgebung [K]/1 -> Add3/1
  PCM_Trigger/1 -> Trigger/2(Trigger)
  T_FinitesVolumen [K]/1 -> Waermeaustausch PCM - Fluid/2(T_FinitesVolumen [K])
  Waermeaustausch PCM - Fluid/2(PQ_PCM_FinitesVolumen [W]) -> PQ_PCM_FinitesVolumen [W]/1
  Waermeaustausch PCM - Umgebung/1(PQ_PCM_Umgebung [W]) -> Add4/1
  Subtract/1 -> Product3/2
  Add5/1 -> Trigger/1(Temp_in)  "T_PCM_k+1 [K]"
  Waermeaustausch PCM - Fluid/1(PQ_PCM_Kuehlfluessigkeit [W]) -> Add4/2
  v_Fahrzeug [m*s^-1]/1 -> Waermeaustausch PCM - Umgebung/3(v_Fahrzeug [m*s^-1])
  Constant16/1 -> Subtract/1
  Delay/1 -> Waermeaustausch PCM - Fluid/1(T_PCM [K]), Waermeaustausch PCM - Umgebung/1(T_PCM [K]), Add5/1, Phasenuebergang/1(Temp), T_PCM [K]/1  "T_PCM_k [K]"
  Product3/1 -> Phasenuebergang/2(dT_in)  "dT_PCM [K]"
  T_PCM_Offset/1 -> Add3/2
  Phasenuebergang/1(dT_out) -> Add5/2
  PV_Kuehlfluessigkeit [m^3*s^-1]/1 -> Waermeaustausch PCM - Fluid/3(PV_PCM [m^3*s^-1])
  T_PCM_init/1 -> Delay/2
  Trigger/2(Trigger_aktiv) -> Phasenuebergang/3(Trigger_aktiv)
